simulink model "scheme5_2"  (R2021a)
settings: Solver=VariableStepAuto  StartTime=0.0  StopTime=30  RelTol=1e-3
values from neighbouring files (symbols this model uses):
  k = 6    [exercise5.m]
  T_1 = 5.1    [exercise5.m]
  T_2 = 0.2    [exercise5.m]
  Td = 0    [exercise5.m]
  Ti = 0.8    [exercise5.m]
undefined symbols (not defined in the file or in its folder): kp
settings Model: Creator=Paweł  LastModifiedBy=Paweł

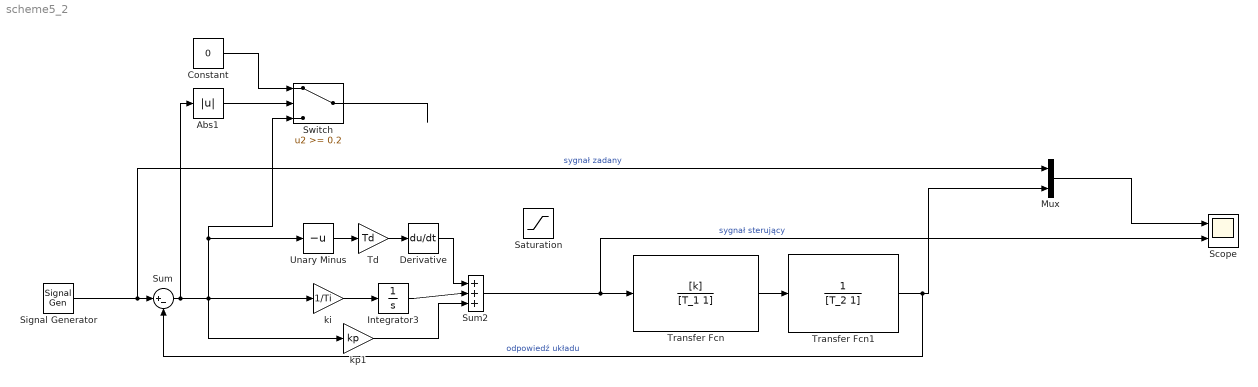
== system scheme5_2 ==
  Abs1 : Abs
  Constant : Constant  Value=0
  Derivative : Derivative
  Integrator3 : Integrator
  Mux : Mux  Inputs=2
  Saturation : Saturate  UpperLimit=2  LowerLimit=-2
  Scope : Scope  NumInputPorts=2
  Signal Generator : SignalGenerator  WaveForm=square  Frequency=0.1
  Sum : Sum  Inputs=|+-
  Sum2 : Sum  Inputs=|+++  SaturateOnIntegerOverflow=on
  Switch : Switch  Threshold=0.2
  Td : Gain  Gain=Td  SaturateOnIntegerOverflow=on  OutDataTypeStr=Inherit: Same as input  ParamDataTypeStr=Inherit: Same as input
  Transfer Fcn : TransferFcn  Numerator=[k]  Denominator=[T_1 1]
  Transfer Fcn1 : TransferFcn  Denominator=[T_2 1]
  Unary Minus : UnaryMinus
  ki : Gain  Gain=1/Ti  SaturateOnIntegerOverflow=on  OutDataTypeStr=Inherit: Same as input  ParamDataTypeStr=Inherit: Same as input
  kp1 : Gain  Gain=kp  SaturateOnIntegerOverflow=on  OutDataTypeStr=Inherit: Same as input  ParamDataTypeStr=Inherit: Same as input
  wires:
  Signal Generator/1 -> Mux/1, Sum/1  "sygnał zadany"
  Transfer Fcn1/1 -> Mux/2, Sum/2  "odpowiedź układu"
  Td/1 -> Derivative/1
  ki/1 -> Integrator3/1
  Transfer Fcn/1 -> Transfer Fcn1/1
  Integrator3/1 -> Sum2/2
  Mux/1 -> Scope/1
  Derivative/1 -> Sum2/1
  Sum/1 -> Abs1/1, ki/1, Unary Minus/1, Switch/3, kp1/1
  Constant/1 -> Switch/1
  Abs1/1 -> Switch/2
  Unary Minus/1 -> Td/1
  kp1/1 -> Sum2/3
  Switch/1 -> ?
  Sum2/1 -> Scope/2, Transfer Fcn/1  "sygnał sterujący"
